simulink model "Speed_LADRC_2018"  (R2023b)
settings: Solver=FixedStepDiscrete  StartTime=0.0  StopTime=10  FixedStep=Ts  MaxStep=1e-6  MinStep=1e-6  RelTol=1e-6
InitFcn:
  | Ts = 5e-7;%仿真步长   2000khz
  | Tpwm = 1e-4;%开关周期
  | Tsample = Tpwm/1;%采样周期/控制周期   除以2就是双采双更，除以1是单采单更
  | Tspeed = 5*Tpwm;%转速采样周期
  | 
  | Pn = 4;%电机极对数
  | Ls = 8.5e-3;%定子电感，采用隐极的，Ld=Lq=Ls
  | Rs = 3;%定子电阻
  | flux = 0.1688;%永磁体磁链
  | Vdc = 311;%直流母线电压
  | J = 0.01;%转动惯量
  | B = 0;%阻尼系数
  | 
  | n_init = 0;%初始转速
  | fc_lpf = 200;%转速计算的低通滤波器截止频率
  | 
  | %转速环PI参数
  | b=1.5*Pn*flux/J;
  | wc=100;
  | wo=200;
  | iqmax=25;
  | %电流环PI参数
  | Ld1 = Ls;
  | Lq1 = Ls;
  | flux1 = flux;
  | Rs1 = Rs;
  | fc = 300;%电流环带宽
  | 
  | Enable = 1;%1代表开启1.5拍延时补偿
  | td=0.00005;
undefined symbols (not defined in the file): DiscIntNeverNeededParam
libraries: slctrl_adaptive x1, spsDCVoltageSourceLib x1, spsPermanentMagnetSynchronousMachineLib x1, simulink x1, spsUniversalBridgeLib x1, sps_lib x1
settings Model: Creator=admin  LastModifiedBy=Lenovo
settings SolverCC: AlgebraicLoopSolver=TrustRegion
settings DataIOCC: ReturnWorkspaceOutputs=off
settings OptimizationCC: ReuseModelBlockBuffer=off
settings DebuggingCC: UnconnectedInputMsg=warning  UnconnectedOutputMsg=warning  UnconnectedLineMsg=warning  ArithmeticOperatorsInVariantConditions=warning
settings ModelReferenceCC: EnableRefExpFcnMdlSchedulingChecks=on
settings SFSimCC: CustomCodeUndefinedFunction=UseInterfaceOnly

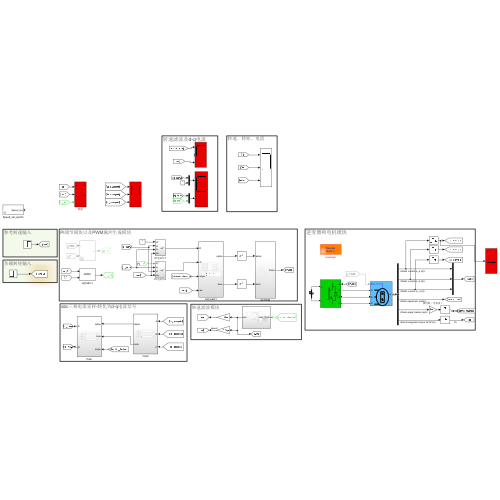
[thumbnail: Simulink's stored preview of the top-level diagram]
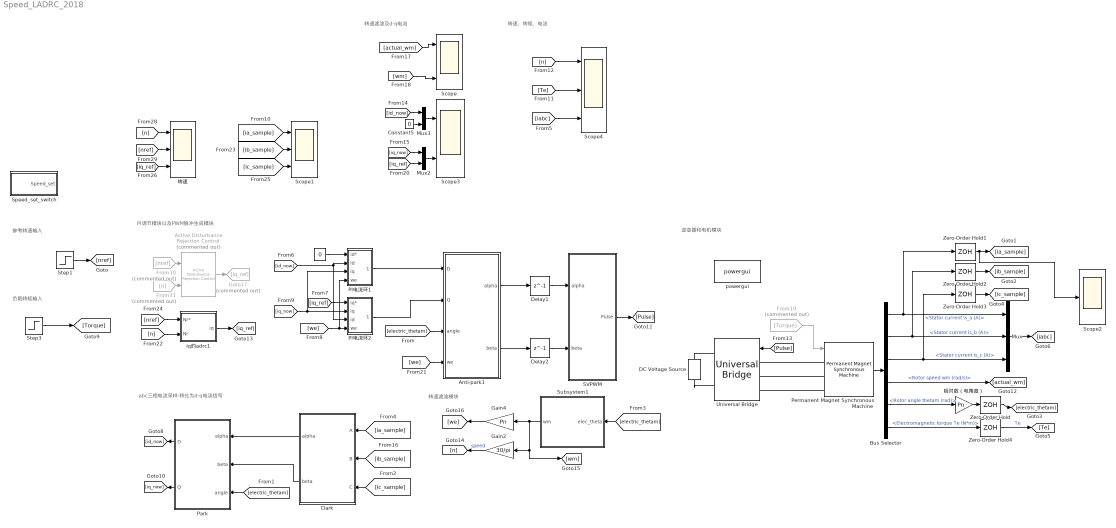
== system Speed_LADRC_2018 ==
  note: 负载转矩输入
  note: PI调节模块以及PWM脉冲生成模块
  note: 逆变器和电机模块
  note: 参考转速输入
  note: abc三相电流采样-转化为d-q电流信号
  note: 转速、转矩、电流
  note: 转速滤波及d-q电流
  note: 转速滤波模块
  " " : Constant  Value=0
  Active Disturbance Rejection Control : slctrl_adaptive/Active Disturbance Rejection Control  Commented=on  time_domain=discrete-time  Ts=0.0001  model_type=first-order  b0=1000  wc=100  wo=1000  x0=0  ulim_checkbox=on  umax=70  umin=-70  xhat_checkbox=off
      settings: LibrarySourceBlock=slctrlblks/Adaptive Control/Active Disturbance Rejection Control
  Anti-park1 : Subsystem
  Bus Selector : BusSelector  OutputSignals=Stator current is_a (A),Stator current is_b (A),Stator current is_c (A),Rotor speed wm (rad/s),Rotor angle thetam (rad),Electromagnetic torque Te (N*m)
  Clark : Subsystem
  Constant5 : Constant  Value=0
  DC Voltage Source : spsDCVoltageSourceLib/DC Voltage Source  Amplitude=Vdc  Measurements=None
  Delay1 : Delay  DelayLength=1  SampleTime=Tpwm
  Delay2 : Delay  DelayLength=1  SampleTime=Tpwm
  From19 : From  Commented=on  GotoTag=Torque
  From30 : From  Commented=on  GotoTag=nref
  From31 : From  Commented=on  GotoTag=n
  Gain2 : Gain  Gain=30/pi
  Gain4 : Gain  Gain=Pn
  Goto17 : Goto  Commented=on  GotoTag=iq_ref
  Mux : Mux  Inputs=3
  Mux2 : Mux  Inputs=2
  Mux3 : Mux  Inputs=2
  PI电流环1 : Subsystem
  PI电流环2 : Subsystem
  "Park " : Subsystem
  Permanent Magnet Synchronous Machine : spsPermanentMagnetSynchronousMachineLib/Permanent Magnet Synchronous Machine  NbPhases=3  FluxDistribution=Sinusoidal  RotorType=Round  MechanicalLoad=Torque Tm  PresetModel=No  ShowDetailedParameters=on  MeasurementBus=off  Resistance=Rs  Inductance=8.5e-3  dqInductances=[0.0009262 0.001024]  La=Ls  MachineConstant=Flux linkage established by magnets (V.s)  Flux=flux  VoltageCst=122.4677  TorqueCst=1.0128  Flat=120  Mechanical=[J B Pn 0]  PolePairs=4  InitialConditions=[n_init/60*2*pi,0, 0,0]  InitialConditions5ph=[0 0 0 0 0 0]  RefAngle=Aligned with phase A axis (original Park)  IterativeDiscreteModel=Trapezoidal non iterative  TsBlock=-1  TsPowergui=0
  SVPWM : Subsystem
  Scope : Scope  NumInputPorts=3
  Scope1 : Scope  NumInputPorts=3
  Scope2 : Scope
  Scope3 : Scope  NumInputPorts=2
  Scope4 : Scope  NumInputPorts=3
  Speed_set_switch : Subsystem  mask{t1=0.3, t2=0.5, t3=0.7, v0=1000, v1=1000, v2=1000, v3=1000}
      mask prompts: t1 "一次速度切换时间/[s]"; t2 "二次速度切换时间/[s]"; t3 "三次速度切换时间/[s]"; v0 "初始速度设定值/[rpm]"; v1 "二次速度设定值/[rpm]"; v2 "三次速度设定值/[rpm]"; v3 "四次速度设定值/[rpm]"
      mask DialogControl DescGroupVar Prompt: Speed Set Switch
      mask DialogControl DescTextVar Prompt: 定时速度切换设置
      mask DialogControl ParameterGroupVar Prompt: 参数
  Step1 : Step  Time=0.25  After=500  SampleTime=0
  Step3 : Step  Time=0.2  After=10  SampleTime=0
  Subsystem1 : Subsystem
  Universal Bridge : spsUniversalBridgeLib/Universal Bridge  Arms=3  SnubberResistance=1e5  SnubberCapacitance=inf  Device=IGBT / Diodes  Ron=1e-3  Lon=0  ForwardVoltages="[  0  0  ]"  ForwardVoltage=0  GTOparameters=[ 10e-6 , 20e-6 ]  IGBTparameters=[ 1e-6 , 2e-6 ]  Measurements=None  Measurements_2=None  converterType=Rectifier
  Zero-Order Hold{,1..4} (5 alike) : ZeroOrderHold  SampleTime=Tsample
  iq的adrc1 : Subsystem
      mask Display: disp('ADRC')
  powergui : sps_lib/powergui  Priority=1  SimulationMode=Discrete  SampleTime=Ts  frequency=60  Iterations=50  frequencyindice=0  Pbase=100e6  ErrMax=1e-4  UnitsV=kV  UnitsW=MW  buscounter=0  FunctionMessages=off  echomessages=off  EnableUseOfTLC=off  CurrentSourceSwitches=off  DisableSnubberDevices=off  DisableRonSwitches=off  DisableVfSwitches=off  DisplayEquations=off  AutomaticDiscreteSolvers=off  SolverType=Tustin/Backward Euler (TBE)  Interpol=off  ExternalGateDelay=off  methode=off  Ts=100  x0status=blocks  SPID=off  SwTol=0  HookPort=off  NonlinearTolerance=1e-4  nMaxIteration=100  ContinueOnMaxIteration=off  RestoreLinks=warning  ResistiveCurrentMeasurement=off  Frange=[0:2:500]  Ylog=off  Xlog=on  ShowGrid=off  save=off  variable=ZData  structure=ScopeData1  ZoomFFT=on  StartTime=0.225  cycles=8  DisplayStyle=1  fundamental=80  FreqAxis=off  MaxFrequency=10000  frequencyindicesteady=1  RmsSteady=1  display=off
  极对数（电角度） : Gain  Gain=Pn
  转速 : Scope  NumInputPorts=3
  wires:
  iq的adrc1/1(iq) -> [iq_ref]
  [nref] -> iq的adrc1/1(Nr*)
  Step1/1 -> [nref]
  Step3/1 -> [Torque]
  [ia_sample] -> Clark/1(A)
  Clark/2(beta) -> "Park "/2(beta)
  [ic_sample] -> Clark/3(C)
  [electric_thetam] -> "Park "/3(angle)
  [ib_sample] -> Clark/2(B)
  "Park "/1(D) -> [id_now]
  Clark/1(alpha) -> "Park "/1(alpha)
  "Park "/2(Q) -> [iq_now]
  [n] -> iq的adrc1/2("Nr ")
  Zero-Order Hold4/1 -> [Te]  "Te"
  Permanent Magnet Synchronous Machine/1 -> Bus Selector/1
  Bus Selector/2 -> Mux/2, Zero-Order Hold2/1  "<Stator current is_b (A)>"
  From19/1 -> Permanent Magnet Synchronous Machine/1
  Zero-Order Hold2/1 -> [ib_sample]
  Zero-Order Hold3/1 -> [ic_sample]
  [Pulse] -> Universal Bridge/1
  Zero-Order Hold/1 -> [electric_thetam]
  Bus Selector/3 -> Mux/3, Zero-Order Hold3/1  "<Stator current is_c (A)>"
  [iq_now] -> PI电流环1/3(iq), PI电流环2/2("iq ")
  Bus Selector/6 -> Zero-Order Hold4/1  "<Electromagnetic torque Te (N*m)>"
  PI电流环1/1("ud* ") -> Anti-park1/1(D)
  [iq_ref] -> PI电流环2/1(iq*)
  Bus Selector/1 -> Mux/1, Zero-Order Hold1/1  "<Stator current is_a (A)>"
  PI电流环2/1("uq* ") -> Anti-park1/2(Q)
  Bus Selector/4 -> [actual_wm]  "<Rotor speed wm (rad/s)>"
  [id_now] -> PI电流环2/3(id), PI电流环1/2(id)
  [electric_thetam] -> Anti-park1/3(angle)
  [we] -> PI电流环1/4(we), PI电流环2/4(we)
  [Te] -> Scope4/2
  Subsystem1/1(wm) -> [wm], Gain2/1, Gain4/1
  Gain4/1 -> [we]
  " "/1 -> PI电流环1/1(id*)
  Mux/1 -> [iabc]
  Gain2/1 -> [n]  "speed"
  [electric_thetam] -> Subsystem1/1(elec_theta)
  Constant5/1 -> Mux3/2
  [n] -> Scope4/1
  Bus Selector/5 -> 极对数（电角度）/1  "<Rotor angle thetam (rad)>"
  Mux3/1 -> Scope3/1
  Mux2/1 -> Scope3/2
  [iq_now] -> Mux2/1
  [id_now] -> Mux3/1
  Zero-Order Hold1/1 -> Scope2/1, [ia_sample]
  [actual_wm] -> Scope/1
  [iq_ref] -> Mux2/2
  极对数（电角度）/1 -> Zero-Order Hold/1
  [wm] -> Scope/3
  [we] -> Anti-park1/4(we)
  Anti-park1/1(alpha) -> Delay1/1
  Anti-park1/2(beta) -> Delay2/1
  SVPWM/1(Pulse) -> [Pulse]
  Delay1/1 -> SVPWM/1(alpha)
  Delay2/1 -> SVPWM/2(beta)
  [iabc] -> Scope4/3
  [ia_sample] -> Scope1/1
  [ib_sample] -> Scope1/2
  [ic_sample] -> Scope1/3
  [n] -> 转速/1
  [nref] -> 转速/2
  From30/1 -> Active Disturbance Rejection Control/1
  From31/1 -> Active Disturbance Rejection Control/2
  Active Disturbance Rejection Control/1 -> Goto17/1
  [iq_ref] -> 转速/3
  connections:
  Permanent Magnet Synchronous Machine/LConn3 -- Universal Bridge/LConn3
  Permanent Magnet Synchronous Machine/LConn1 -- Universal Bridge/LConn1
  Permanent Magnet Synchronous Machine/LConn2 -- Universal Bridge/LConn2
  DC Voltage Source/LConn1 -- Universal Bridge/RConn2
  Universal Bridge/RConn1 -- DC Voltage Source/RConn1

== system Speed_LADRC_2018/Anti-park1 ==
  note: 延时触发模块
  note: 坐标变换+1.5拍延时补偿模块
  D : Inport
  Q : Inport  Port=2
  angle : Inport  Port=3
  we : Inport  Port=4
  Constant : Constant  Value=Tpwm
  Constant1 : Constant  Value=Enable
  MATLAB Function : MATLAB Function  TreatAsAtomicUnit=on
  Scope : Scope
  alpha : Outport  VectorParamsAs1DForOutWhenUnconnected=off
  beta : Outport  Port=2  VectorParamsAs1DForOutWhenUnconnected=off
  wires:
  D/1 -> MATLAB Function/1(ud)
  Q/1 -> MATLAB Function/2(uq)
  we/1 -> MATLAB Function/3(we)
  Constant/1 -> MATLAB Function/4(Ts)
  angle/1 -> MATLAB Function/5(theta)
  MATLAB Function/2(ub_ref) -> beta/1
  MATLAB Function/1(ua_ref) -> alpha/1
  Constant1/1 -> MATLAB Function/6(Enable)
  MATLAB Function/3(m) -> Scope/1

== system Speed_LADRC_2018/Clark ==
  A : Inport
  B : Inport  Port=2
  C : Inport  Port=3
  Fcn1 : Fcn  Expr=sqrt(3)/3*(u(2)-u(3))
  Fcn2 : Fcn  Expr=(2/3)*(u(1)-0.5*u(2)-0.5*u(3))
  Mux2 : Mux  Inputs=3
  alpha : Outport  VectorParamsAs1DForOutWhenUnconnected=off
  beta : Outport  Port=2  VectorParamsAs1DForOutWhenUnconnected=off
  wires:
  C/1 -> Mux2/3
  Fcn2/1 -> alpha/1
  Fcn1/1 -> beta/1
  A/1 -> Mux2/1
  B/1 -> Mux2/2
  Mux2/1 -> Fcn1/1, Fcn2/1

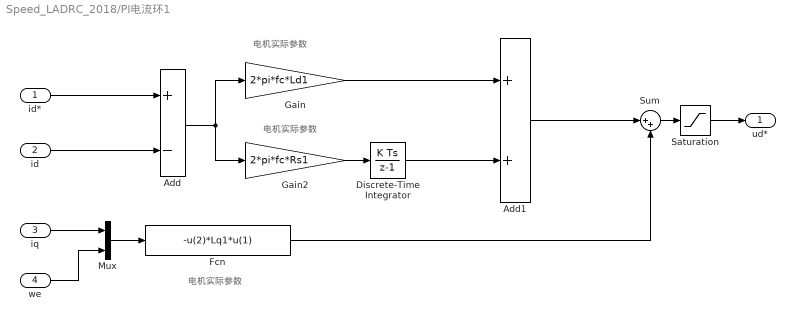
== system Speed_LADRC_2018/PI电流环1 ==
  note: 电机实际参数
  note: 电机实际参数
  note: 电机实际参数
  id* : Inport
  id : Inport  Port=2
  iq : Inport  Port=3
  we : Inport  Port=4
  Add : Sum  Inputs=+-
  Add1 : Sum
  Discrete-Time Integrator : DiscreteIntegrator  SampleTime=Tsample  LimitOutput=on  UpperSaturationLimit=Vdc/sqrt(3)  LowerSaturationLimit=-Vdc/sqrt(3)  ICPrevOutput=DiscIntNeverNeededParam  ICPrevScaledInput=DiscIntNeverNeededParam
  Fcn : Fcn  Expr=-u(2)*Lq1*u(1)
  Gain : Gain  Gain=2*pi*fc*Ld1
  Gain2 : Gain  Gain=2*pi*fc*Rs1
  Mux : Mux  Inputs=2
  Saturation : Saturate  UpperLimit=Vdc/sqrt(3)  LowerLimit=-Vdc/sqrt(3)
  Sum : Sum  Inputs=|++
  "ud* " : Outport  VectorParamsAs1DForOutWhenUnconnected=off
  wires:
  we/1 -> Mux/2
  iq/1 -> Mux/1
  id*/1 -> Add/1
  id/1 -> Add/2
  Mux/1 -> Fcn/1
  Add1/1 -> Sum/1
  Fcn/1 -> Sum/2
  Sum/1 -> Saturation/1
  Saturation/1 -> "ud* "/1
  Gain/1 -> Add1/1
  Gain2/1 -> Discrete-Time Integrator/1
  Discrete-Time Integrator/1 -> Add1/2
  Add/1 -> Gain2/1, Gain/1

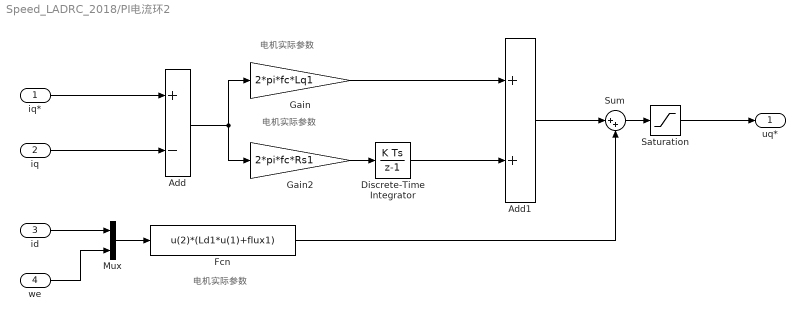
== system Speed_LADRC_2018/PI电流环2 ==
  note: 电机实际参数
  note: 电机实际参数
  note: 电机实际参数
  iq* : Inport
  "iq " : Inport  Port=2
  id : Inport  Port=3
  we : Inport  Port=4
  Add : Sum  Inputs=+-
  Add1 : Sum
  Discrete-Time Integrator : DiscreteIntegrator  SampleTime=Tsample  LimitOutput=on  UpperSaturationLimit=Vdc/sqrt(3)  LowerSaturationLimit=-Vdc/sqrt(3)  ICPrevOutput=DiscIntNeverNeededParam  ICPrevScaledInput=DiscIntNeverNeededParam
  Fcn : Fcn  Expr=u(2)*(Ld1*u(1)+flux1)
  Gain : Gain  Gain=2*pi*fc*Lq1
  Gain2 : Gain  Gain=2*pi*fc*Rs1
  Mux : Mux  Inputs=2
  Saturation : Saturate  UpperLimit=Vdc/sqrt(3)  LowerLimit=-Vdc/sqrt(3)  LinearizeAsGain=off
  Sum : Sum  Inputs=|++
  "uq* " : Outport  VectorParamsAs1DForOutWhenUnconnected=off
  wires:
  id/1 -> Mux/1
  we/1 -> Mux/2
  "iq "/1 -> Add/2
  iq*/1 -> Add/1
  Mux/1 -> Fcn/1
  Add/1 -> Gain/1, Gain2/1
  Add1/1 -> Sum/1
  Gain2/1 -> Discrete-Time Integrator/1
  Discrete-Time Integrator/1 -> Add1/2
  Gain/1 -> Add1/1
  Fcn/1 -> Sum/2
  Sum/1 -> Saturation/1
  Saturation/1 -> "uq* "/1

== system Speed_LADRC_2018/Park  ==
  alpha : Inport
  beta : Inport  Port=2
  angle : Inport  Port=3
  Fcn1 : Fcn  Expr=-sin(u(3))*u(1)+cos(u(3))*u(2)
  Fcn2 : Fcn  Expr=cos(u(3))*u(1)+sin(u(3))*u(2)
  Mux2 : Mux  Inputs=3
  D : Outport  VectorParamsAs1DForOutWhenUnconnected=off
  Q : Outport  Port=2  VectorParamsAs1DForOutWhenUnconnected=off
  wires:
  angle/1 -> Mux2/3
  Mux2/1 -> Fcn2/1, Fcn1/1
  Fcn2/1 -> D/1
  Fcn1/1 -> Q/1
  alpha/1 -> Mux2/1
  beta/1 -> Mux2/2

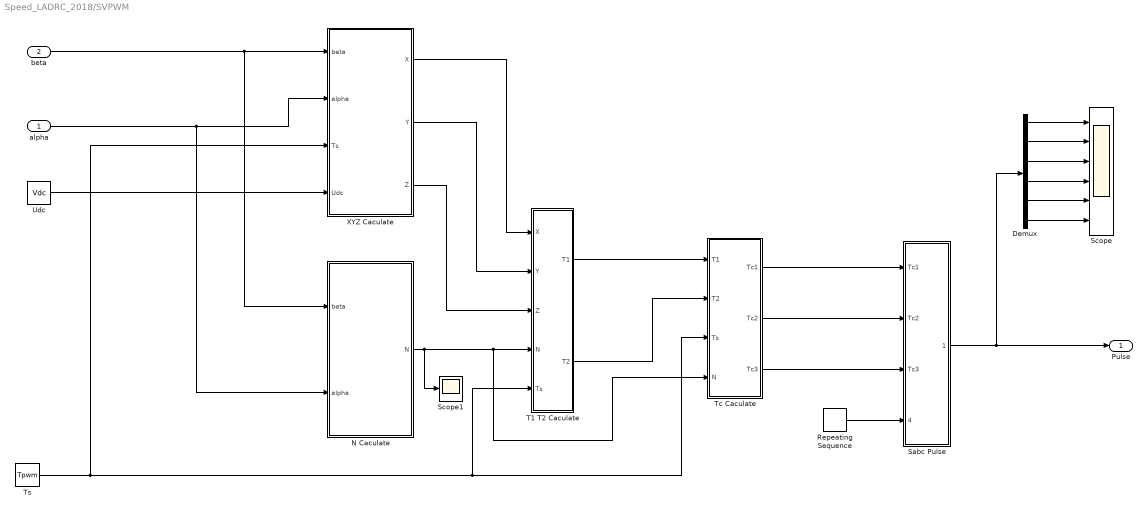
== system Speed_LADRC_2018/SVPWM ==
  alpha : Inport
  beta : Inport  Port=2
  Demux : Demux  Outputs=6
  N Caculate : Subsystem
  Repeating Sequence : simulink/Sources/Repeating Sequence  rep_seq_t=[0 0.5*Tpwm Tpwm]  rep_seq_y=[0 0.5*Tpwm 0]
  Sabc Pulse : Subsystem
  Scope : Scope  NumInputPorts=6
  Scope1 : Scope
  T1 T2 Caculate : Subsystem
  Tc Caculate : Subsystem
  Ts : Constant  Value=Tpwm
  "Udc " : Constant  Value=Vdc
  XYZ Caculate : Subsystem
  Pulse : Outport  VectorParamsAs1DForOutWhenUnconnected=off
  wires:
  beta/1 -> N Caculate/1(beta), XYZ Caculate/1(beta)
  alpha/1 -> N Caculate/2(alpha), XYZ Caculate/2(alpha)
  XYZ Caculate/1(X) -> T1 T2 Caculate/1(X)
  XYZ Caculate/2(Y) -> T1 T2 Caculate/2(Y)
  XYZ Caculate/3(Z) -> T1 T2 Caculate/3(Z)
  N Caculate/1(N) -> Scope1/1, Tc Caculate/4(N), T1 T2 Caculate/4(N)
  Ts/1 -> XYZ Caculate/3("Ts "), Tc Caculate/3(Ts), T1 T2 Caculate/5("Ts ")
  T1 T2 Caculate/1(T1) -> Tc Caculate/1(T1)
  T1 T2 Caculate/2(T2) -> Tc Caculate/2(T2)
  Tc Caculate/1(Tc1) -> Sabc Pulse/1(Tc1)
  Tc Caculate/2(Tc2) -> Sabc Pulse/2(Tc2)
  Tc Caculate/3(Tc3) -> Sabc Pulse/3(Tc3)
  Sabc Pulse/1("Pulse ") -> Demux/1, Pulse/1
  "Udc "/1 -> XYZ Caculate/4(Udc)
  Repeating Sequence/1 -> Sabc Pulse/4(Wave)
  Demux/1 -> Scope/1
  Demux/2 -> Scope/2
  Demux/3 -> Scope/3
  Demux/4 -> Scope/4
  Demux/5 -> Scope/5
  Demux/6 -> Scope/6

== system Speed_LADRC_2018/Speed_set_switch ==
  Clock2 : Clock
  MATLAB Function2 : MATLAB Function  TreatAsAtomicUnit=on
  Step : Step  Time=t1  Before=v0  After=v1  SampleTime=0
  Step1 : Step  Time=t2  Before=v1  After=v2  SampleTime=0
  Step2 : Step  Time=t3  Before=v2  After=v3  SampleTime=0
  t : Constant  Value=t1
  t. : Constant  Value=t2
  tt : Constant  Value=t3
  v : Constant  Value=v0
  Speed_set : Outport  VectorParamsAs1DForOutWhenUnconnected=off
  wires:
  MATLAB Function2/1(y) -> Speed_set/1
  Clock2/1 -> MATLAB Function2/1(t)
  Step/1 -> MATLAB Function2/5(u1)  "v1"
  t/1 -> MATLAB Function2/2(t1)
  Step1/1 -> MATLAB Function2/6(u2)  "v2"
  t./1 -> MATLAB Function2/3(t2)
  v/1 -> MATLAB Function2/8(v0)
  tt/1 -> MATLAB Function2/4(t3)
  Step2/1 -> MATLAB Function2/7(u3)

== system Speed_LADRC_2018/Subsystem1 ==
  note: 转速初始值
  note: 低通滤波器截止频率
  elec_theta : Inport
  Add2 : Sum
  Clock : Clock
  Constant : Constant  Value=n_init
  Constant1 : Constant  Value=fc_lpf
  Constant2 : Constant  Value=Tsample
  Delay3 : Delay  DelayLength=1
  Delay4 : Delay  DelayLength=1
  MATLAB Function2 : MATLAB Function  TreatAsAtomicUnit=on
  Zero-Order Hold1 : ZeroOrderHold  SampleTime=Tsample
  Zero-Order Hold6 : ZeroOrderHold  SampleTime=Tsample
  实际噪声模拟 : RandomNumber  Mean=0.00000000125  Variance=0.00000000125  SampleTime=Tsample
  极对数 : Gain  Gain=1/Pn
  wm : Outport  VectorParamsAs1DForOutWhenUnconnected=off
  wires:
  MATLAB Function2/1(wm_now) -> wm/1, Delay4/1
  elec_theta/1 -> 极对数/1
  Add2/1 -> Delay3/1, MATLAB Function2/1(thetam)
  Delay4/1 -> MATLAB Function2/4(wm_1)
  极对数/1 -> Zero-Order Hold6/1
  Zero-Order Hold6/1 -> Add2/1
  Delay3/1 -> MATLAB Function2/2(thetamk1)
  Constant2/1 -> MATLAB Function2/3(Tsample)
  实际噪声模拟/1 -> Add2/2
  Constant/1 -> MATLAB Function2/5(n_init)
  Zero-Order Hold1/1 -> MATLAB Function2/6(t)
  Clock/1 -> Zero-Order Hold1/1
  Constant1/1 -> MATLAB Function2/7(fc_lpf)

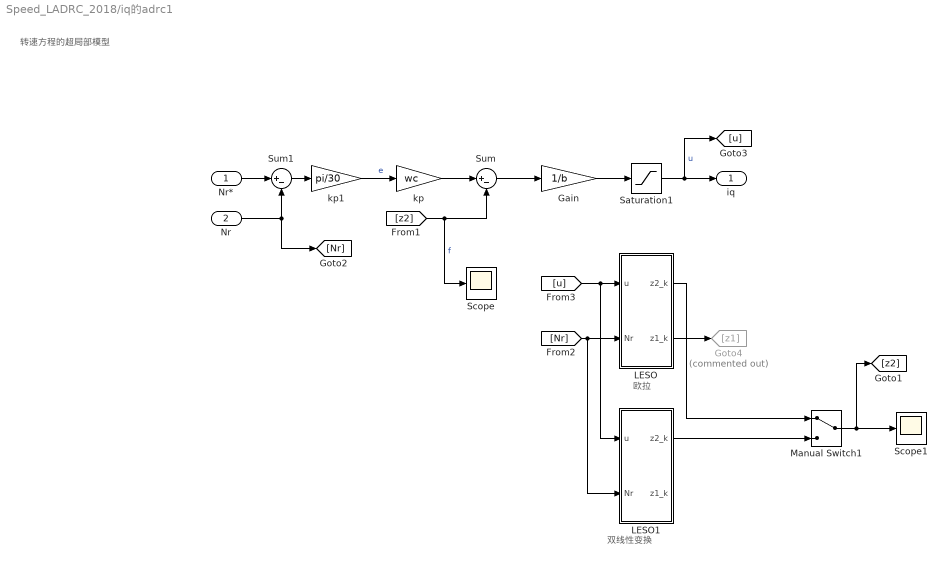
== system Speed_LADRC_2018/iq的adrc1 ==
  note: 双线性变换
  note: 转速方程的超局部模型
  note: 欧拉
  Nr* : Inport
  "Nr " : Inport  Port=2
  Gain : Gain  Gain=1/b
  Goto4 : Goto  Commented=on  GotoTag=z1
  LESO : Subsystem
  LESO1 : Subsystem
  Manual Switch1 : ManualSwitch
  Saturation1 : Saturate  UpperLimit=iqmax  LowerLimit=-iqmax
  Scope : Scope
  Scope1 : Scope
  Sum : Sum  Inputs=|+-
  Sum1 : Sum  Inputs=|+-
  kp : Gain  Gain=wc
  kp1 : Gain  Gain=pi/30
  iq : Outport
  wires:
  kp/1 -> Sum/1
  Nr*/1 -> Sum1/1
  Saturation1/1 -> [u], iq/1  "u"
  Gain/1 -> Saturation1/1
  Sum1/1 -> kp1/1
  LESO/1(z2_k) -> Manual Switch1/1
  [Nr] -> LESO/2("Nr "), LESO1/2("Nr ")
  [z2] -> Sum/2, Scope/1  "f"
  "Nr "/1 -> [Nr], Sum1/2
  Sum/1 -> Gain/1
  [u] -> LESO1/1(u), LESO/1(u)
  kp1/1 -> kp/1  "e"
  LESO/2(z1_k) -> Goto4/1
  Manual Switch1/1 -> [z2], Scope1/1
  LESO1/1(z2_k) -> Manual Switch1/2

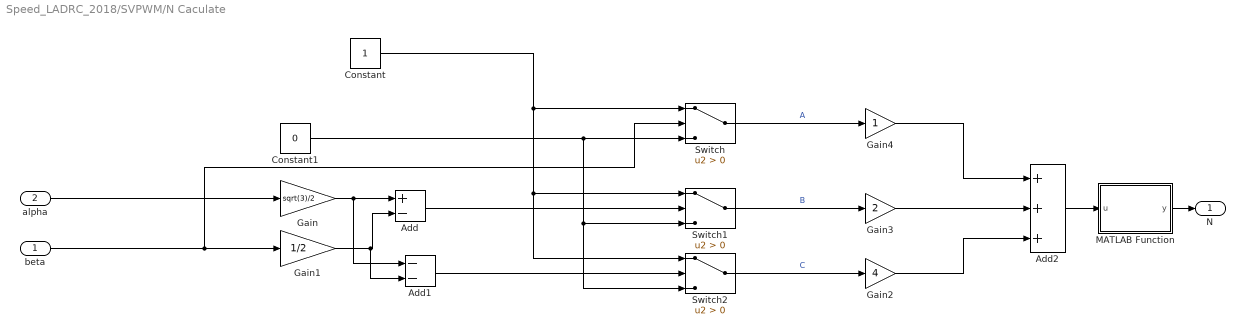
== system Speed_LADRC_2018/SVPWM/N Caculate ==
  beta : Inport
  alpha : Inport  Port=2
  Add : Sum  Inputs=+-
  Add1 : Sum  Inputs=--
  Add2 : Sum  Inputs=+++
  Constant : Constant
  Constant1 : Constant  Value=0
  Gain : Gain  Gain=sqrt(3)/2
  Gain1 : Gain  Gain=1/2
  Gain2 : Gain  Gain=4
  Gain3 : Gain  Gain=2
  Gain4 : Gain
  MATLAB Function : MATLAB Function  TreatAsAtomicUnit=on
  Switch : Switch  Criteria=u2 > Threshold  SaturateOnIntegerOverflow=off  InputSameDT=off
  Switch1 : Switch  Criteria=u2 > Threshold  SaturateOnIntegerOverflow=off  InputSameDT=off
  Switch2 : Switch  Criteria=u2 > Threshold  SaturateOnIntegerOverflow=off  InputSameDT=off
  N : Outport  VectorParamsAs1DForOutWhenUnconnected=off
  wires:
  Switch/1 -> Gain4/1  "A"
  Add/1 -> Switch1/2
  Gain/1 -> Add1/1, Add/1
  Gain3/1 -> Add2/2
  Gain2/1 -> Add2/3
  Constant/1 -> Switch/1, Switch2/1, Switch1/1
  Add1/1 -> Switch2/2
  Gain1/1 -> Add1/2, Add/2
  Add2/1 -> MATLAB Function/1(u)
  Constant1/1 -> Switch2/3, Switch1/3, Switch/3
  Gain4/1 -> Add2/1
  beta/1 -> Switch/2, Gain1/1
  Switch2/1 -> Gain2/1  "C"
  Switch1/1 -> Gain3/1  "B"
  alpha/1 -> Gain/1
  MATLAB Function/1(y) -> N/1

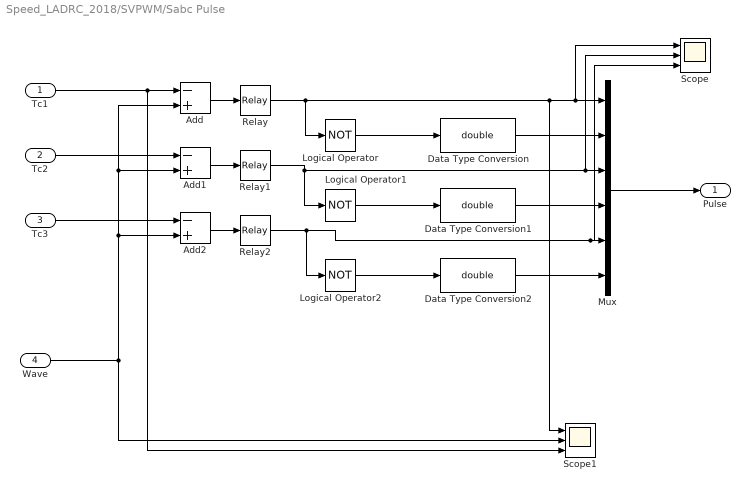
== system Speed_LADRC_2018/SVPWM/Sabc Pulse ==
  Tc1 : Inport
  Tc2 : Inport  Port=2
  Tc3 : Inport  Port=3
  Wave : Inport  Port=4
  Add : Sum  Inputs=-+
  Add1 : Sum  Inputs=-+
  Add2 : Sum  Inputs=-+
  Data Type Conversion : DataTypeConversion  OutDataTypeStr=double  SaturateOnIntegerOverflow=off  RndMeth=Floor
  Data Type Conversion1 : DataTypeConversion  OutDataTypeStr=double  SaturateOnIntegerOverflow=off  RndMeth=Floor
  Data Type Conversion2 : DataTypeConversion  OutDataTypeStr=double  SaturateOnIntegerOverflow=off  RndMeth=Floor
  Logical Operator : Logic  Operator=NOT  AllPortsSameDT=off  OutDataTypeStr=boolean
  Logical Operator1 : Logic  Operator=NOT  AllPortsSameDT=off  OutDataTypeStr=boolean
  Logical Operator2 : Logic  Operator=NOT  AllPortsSameDT=off  OutDataTypeStr=boolean
  Mux : Mux  Inputs=6
  Relay : Relay
  Relay1 : Relay
  Relay2 : Relay
  Scope : Scope  NumInputPorts=3
  Scope1 : Scope  NumInputPorts=3
  "Pulse " : Outport  VectorParamsAs1DForOutWhenUnconnected=off
  wires:
  Add/1 -> Relay/1
  Add1/1 -> Relay1/1
  Wave/1 -> Add2/2, Add1/2, Add/2, Scope1/2
  Tc2/1 -> Add1/1
  Tc1/1 -> Scope1/3, Add/1
  Tc3/1 -> Add2/1
  Logical Operator/1 -> Data Type Conversion/1
  Logical Operator1/1 -> Data Type Conversion1/1
  Add2/1 -> Relay2/1
  Logical Operator2/1 -> Data Type Conversion2/1
  Mux/1 -> "Pulse "/1
  Relay/1 -> Scope1/1, Scope/1, Mux/1, Logical Operator/1
  Relay1/1 -> Scope/2, Mux/3, Logical Operator1/1
  Relay2/1 -> Logical Operator2/1, Scope/3, Mux/5
  Data Type Conversion/1 -> Mux/2
  Data Type Conversion1/1 -> Mux/4
  Data Type Conversion2/1 -> Mux/6

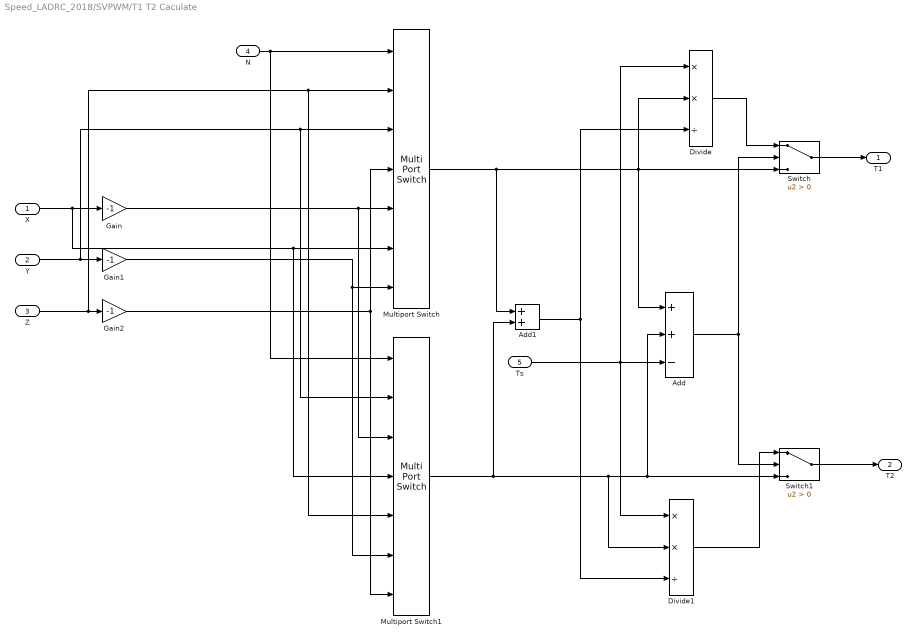
== system Speed_LADRC_2018/SVPWM/T1 T2 Caculate ==
  X : Inport
  Y : Inport  Port=2
  Z : Inport  Port=3
  N : Inport  Port=4
  "Ts " : Inport  Port=5
  Add : Sum  Inputs=++-
  Add1 : Sum
  Divide : Product  Inputs=**/
  Divide1 : Product  Inputs=**/
  Gain : Gain  Gain=-1
  Gain1 : Gain  Gain=-1
  Gain2 : Gain  Gain=-1
  Multiport Switch : MultiPortSwitch  Inputs=6  SaturateOnIntegerOverflow=off  InputSameDT=off
  Multiport Switch1 : MultiPortSwitch  Inputs=6  SaturateOnIntegerOverflow=off  InputSameDT=off
  Switch : Switch  Criteria=u2 > Threshold  SaturateOnIntegerOverflow=off  InputSameDT=off
  Switch1 : Switch  Criteria=u2 > Threshold  SaturateOnIntegerOverflow=off  InputSameDT=off
  T1 : Outport  VectorParamsAs1DForOutWhenUnconnected=off
  T2 : Outport  Port=2  VectorParamsAs1DForOutWhenUnconnected=off
  wires:
  Y/1 -> Multiport Switch1/2, Multiport Switch/3, Gain1/1
  X/1 -> Multiport Switch1/4, Multiport Switch/6, Gain/1
  N/1 -> Multiport Switch/1, Multiport Switch1/1
  Z/1 -> Multiport Switch1/5, Multiport Switch/2, Gain2/1
  Gain2/1 -> Multiport Switch1/7, Multiport Switch/4
  Gain/1 -> Multiport Switch1/3, Multiport Switch/5
  Gain1/1 -> Multiport Switch1/6, Multiport Switch/7
  Multiport Switch/1 -> Add1/1, Divide/2, Add/1, Switch/3
  Multiport Switch1/1 -> Add1/2, Divide1/2, Add/2, Switch1/3
  "Ts "/1 -> Divide1/1, Divide/1, Add/3
  Add/1 -> Switch1/2, Switch/2
  Divide/1 -> Switch/1
  Add1/1 -> Divide/3, Divide1/3
  Switch/1 -> T1/1
  Switch1/1 -> T2/1
  Divide1/1 -> Switch1/1

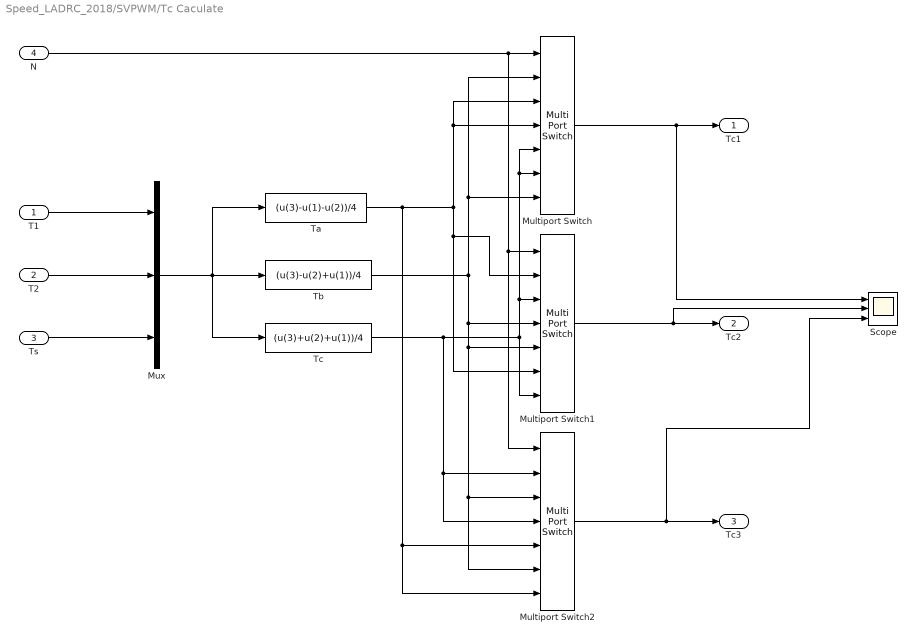
== system Speed_LADRC_2018/SVPWM/Tc Caculate ==
  T1 : Inport
  T2 : Inport  Port=2
  Ts : Inport  Port=3
  N : Inport  Port=4
  Multiport Switch : MultiPortSwitch  Inputs=6  SaturateOnIntegerOverflow=off  InputSameDT=off
  Multiport Switch1 : MultiPortSwitch  Inputs=6  SaturateOnIntegerOverflow=off  InputSameDT=off
  Multiport Switch2 : MultiPortSwitch  Inputs=6  SaturateOnIntegerOverflow=off  InputSameDT=off
  Mux : Mux  Inputs=3
  Scope : Scope  NumInputPorts=3
  Ta : Fcn  Expr=(u(3)-u(1)-u(2))/4
  Tb : Fcn  Expr=(u(3)-u(2)+u(1))/4
  Tc : Fcn  Expr=(u(3)+u(2)+u(1))/4
  Tc1 : Outport  VectorParamsAs1DForOutWhenUnconnected=off
  Tc2 : Outport  Port=2  VectorParamsAs1DForOutWhenUnconnected=off
  Tc3 : Outport  Port=3  VectorParamsAs1DForOutWhenUnconnected=off
  wires:
  T2/1 -> Mux/2
  T1/1 -> Mux/1
  Ts/1 -> Mux/3
  Mux/1 -> Tc/1, Ta/1, Tb/1
  N/1 -> Multiport Switch2/1, Multiport Switch1/1, Multiport Switch/1
  Ta/1 -> Multiport Switch2/7, Multiport Switch2/5, Multiport Switch/3, Multiport Switch/4, Multiport Switch1/6, Multiport Switch1/2
  Tb/1 -> Multiport Switch/7, Multiport Switch/2, Multiport Switch1/4, Multiport Switch2/6, Multiport Switch2/3, Multiport Switch1/5
  Tc/1 -> Multiport Switch2/4, Multiport Switch2/2, Multiport Switch1/7, Multiport Switch1/3, Multiport Switch/6, Multiport Switch/5
  Multiport Switch/1 -> Scope/1, Tc1/1
  Multiport Switch1/1 -> Scope/2, Tc2/1
  Multiport Switch2/1 -> Scope/3, Tc3/1

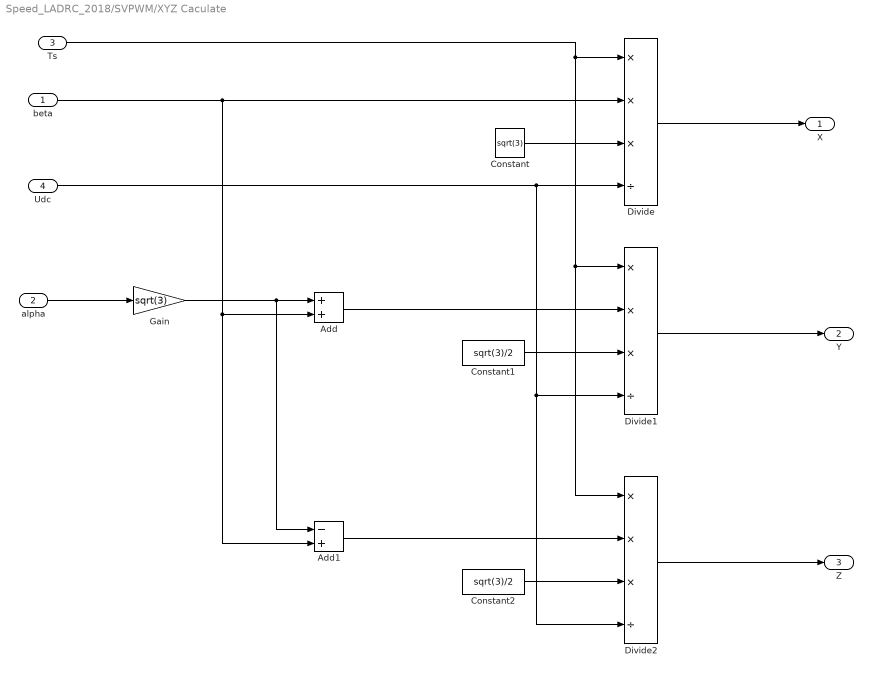
== system Speed_LADRC_2018/SVPWM/XYZ Caculate ==
  beta : Inport
  alpha : Inport  Port=2
  "Ts " : Inport  Port=3
  Udc : Inport  Port=4
  Add : Sum
  Add1 : Sum  Inputs=-+
  Constant : Constant  Value=sqrt(3)
  Constant1 : Constant  Value=sqrt(3)/2
  Constant2 : Constant  Value=sqrt(3)/2
  Divide : Product  Inputs=***/
  Divide1 : Product  Inputs=***/
  Divide2 : Product  Inputs=***/
  Gain : Gain  Gain=sqrt(3)
  X : Outport  VectorParamsAs1DForOutWhenUnconnected=off
  Y : Outport  Port=2  VectorParamsAs1DForOutWhenUnconnected=off
  Z : Outport  Port=3  VectorParamsAs1DForOutWhenUnconnected=off
  wires:
  "Ts "/1 -> Divide2/1, Divide1/1, Divide/1
  Udc/1 -> Divide1/4, Divide2/4, Divide/4
  Constant/1 -> Divide/3
  beta/1 -> Add1/2, Add/2, Divide/2
  Constant2/1 -> Divide2/3
  Constant1/1 -> Divide1/3
  Add/1 -> Divide1/2
  Add1/1 -> Divide2/2
  Gain/1 -> Add1/1, Add/1
  alpha/1 -> Gain/1
  Divide1/1 -> Y/1
  Divide/1 -> X/1
  Divide2/1 -> Z/1

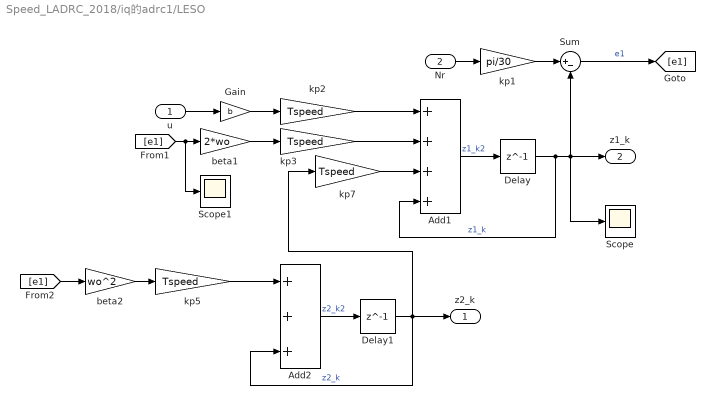
== system Speed_LADRC_2018/iq的adrc1/LESO ==
  u : Inport
  "Nr " : Inport  Port=2
  Add1 : Sum  Inputs=++++
  Add2 : Sum  Inputs=+++
  Delay : Delay  DelayLength=1  SampleTime=Tspeed
  Delay1 : Delay  DelayLength=1  SampleTime=Tspeed
  Gain : Gain  Gain=b
  Scope : Scope
  Scope1 : Scope
  Sum : Sum  Inputs=|+-
  beta1 : Gain  Gain=2*wo
  beta2 : Gain  Gain=wo^2
  kp1 : Gain  Gain=pi/30
  kp{2..3,5,7} (4 alike) : Gain  Gain=Tspeed
  z2_k : Outport  VectorParamsAs1DForOutWhenUnconnected=off
  z1_k : Outport  Port=2  VectorParamsAs1DForOutWhenUnconnected=off
  wires:
  "Nr "/1 -> kp1/1
  u/1 -> Gain/1
  Add1/1 -> Delay/1  "z1_k2"
  Gain/1 -> kp2/1
  kp2/1 -> Add1/1
  kp3/1 -> Add1/2
  Delay1/1 -> kp7/1, z2_k/1, Add2/3  "z2_k"
  Add2/1 -> Delay1/1  "z2_k2"
  kp5/1 -> Add2/1
  [e1] -> Scope1/1, beta1/1
  beta1/1 -> kp3/1
  [e1] -> beta2/1
  beta2/1 -> kp5/1
  Delay/1 -> Add1/4, Sum/2, Scope/1, z1_k/1  "z1_k"
  Sum/1 -> [e1]  "e1"
  kp1/1 -> Sum/1
  kp7/1 -> Add1/3

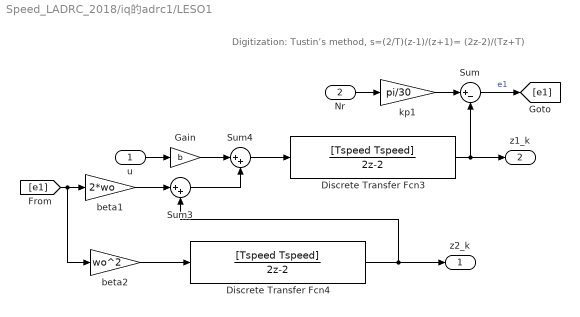
== system Speed_LADRC_2018/iq的adrc1/LESO1 ==
  note: Digitization: Tustin’s method, s=(2/T)(z-1)/(z+1)= (2z-2)/(Tz+T)
  u : Inport
  "Nr " : Inport  Port=2
  Discrete Transfer Fcn3 : DiscreteTransferFcn  Numerator=[Tspeed Tspeed]  Denominator=[2 -2]  SampleTime=Tspeed
  Discrete Transfer Fcn4 : DiscreteTransferFcn  Numerator=[Tspeed Tspeed]  Denominator=[2 -2]  SampleTime=Tspeed
  Gain : Gain  Gain=b
  Sum : Sum  Inputs=|+-
  Sum3 : Sum  Inputs=|++
  Sum4 : Sum  Inputs=|++
  beta1 : Gain  Gain=2*wo
  beta2 : Gain  Gain=wo^2
  kp1 : Gain  Gain=pi/30
  z2_k : Outport  VectorParamsAs1DForOutWhenUnconnected=off
  z1_k : Outport  Port=2  VectorParamsAs1DForOutWhenUnconnected=off
  wires:
  beta1/1 -> Sum3/1
  Gain/1 -> Sum4/1
  kp1/1 -> Sum/1
  Sum/1 -> [e1]  "e1"
  u/1 -> Gain/1
  "Nr "/1 -> kp1/1
  beta2/1 -> Discrete Transfer Fcn4/1
  Sum3/1 -> Sum4/2
  Sum4/1 -> Discrete Transfer Fcn3/1
  Discrete Transfer Fcn3/1 -> Sum/2, z1_k/1
  Discrete Transfer Fcn4/1 -> Sum3/2, z2_k/1
  [e1] -> beta2/1, beta1/1

== matlab function Speed_LADRC_2018/Subsystem1/MATLAB Function2 ==
  data: thetam input; wm_now output; thetamk1 input; Tsample input; wm_1 input; n_init input; t input; fc_lpf input
function wm_now = fcn(thetam,thetamk1,Tsample,wm_1,n_init,t,fc_lpf)

wm = (thetam-thetamk1)/Tsample;
    
%离散化低通滤波器的参考网站：
%https://blog.csdn.net/wanrenqi/article/details/105559070?ops_request_misc=%257B%2522request%255Fid%2522%253A%25221EC2FA41-AB73-4B59-BC31-7DD0178B5C6C%2522%252C%2522scm%2522%253A%252220140713.130102334..%2522%257D&request_id=1EC2FA41-AB73-4B59-BC31-7DD0178B5C6C&biz_id=0&utm_medium=distribute.pc_search_result.none-task-blog-2~all~sobaiduend~default-1-105559070-null-null.142^v100^pc_search_result_base6&utm_term=%E4%BD%8E%E9%80%9A%E6%BB%A4%E6%B3%A2%E5%99%A8%E7%A6%BB%E6%95%A3%E5%8C%96&spm=1018.2226.3001.4187
%选择低通滤波器截止频率为fc_lpf，所以可以计算出下列的低通滤波系数

low_pass_factor1 = 2*pi*fc_lpf*Tsample;
low_pass_factor2 = low_pass_factor1/(1+low_pass_factor1);

%离散化的低通滤波器的表达式
wm_now = low_pass_factor2*wm+(1-low_pass_factor2)*wm_1;

if t==0
    wm_now = n_init/60*2*pi;
end

end

== matlab function Speed_LADRC_2018/SVPWM/N Caculate/MATLAB Function ==
  data: u input; y output
function y = fcn(u)
if u==0
    y=1;
else
    y = u;
end

== matlab function Speed_LADRC_2018/Anti-park1/MATLAB Function ==
  data: ud input; ua_ref output; uq input; we input; Ts input; ub_ref output; theta input; Enable input; m output
function [ua_ref,ub_ref,m] = fcn(ud,uq,we,Ts,theta,Enable)
%这个模块是1.5拍延时补偿环节。
%转速越高的话，延时对电机的影响越大。

m = 2/(we*Ts)*(sin(0.5*we*Ts));
theta_delay = theta+1.5*we*Ts;
if (we == 0)||(Enable == 0) %%如果we等于0的话，上面的m无法计算。
   m = 1; 
   theta_delay = theta;
end


ua_ref = m*(cos(theta_delay)*ud - sin(theta_delay)*uq);
ub_ref = m*(sin(theta_delay)*ud + cos(theta_delay)*uq);

end

== matlab function Speed_LADRC_2018/Speed_set_switch/MATLAB Function2 ==
  data: t input; t1 input; t2 input; t3 input; y output; u1 input; u2 input; u3 input; v0 input
function y = fcn(t, t1,t2,t3,u1,u2,u3,v0)

if t<t1
    y=v0;
elseif t>t1 && t<t2
    y = u1;
elseif t>t2 && t<t3
    y = u2;
else 
    y = u3;

    
end
